simulink model "DataloggerUDP"  (R2015a)
settings: Solver=FixedStepDiscrete  SolverMode=SingleTasking  StartTime=0.0  StopTime=10.0  FixedStep=1e-3  RelTol=1e-3
libraries: mbed_ethernet_udp x3, mbed_lib x2, simulink x1
settings Model: Creator=oh  LastModifiedBy=oh
settings OptimizationCC: OptimizeModelRefInitCode=on  LifeSpan=1
settings HardwareCC: ProdLargestAtomicInteger=Long  ProdLargestAtomicFloat=Double  ProdEndianess=LittleEndian  ProdHWDeviceType=ARM Compatible->ARM Cortex
settings RTWCC: SystemTargetFile=mbed.tlc  TemplateMakefile=mbed.tmf  Description=Mbed Target (Embedded Target)  TargetLang=C++
settings CodeAppCC: IgnoreCustomStorageClasses=off
settings STFCustomTargetCC: CombineOutputUpdateFcns=on  SupportContinuousTime=off  SupportVariableSizeSignals=off  SystemTargetFile=mbed.tlc
settings ERTTargetCC: SupportContinuousTime=off  SupportVariableSizeSignals=off  ERTCustomFileTemplate=mbed_file_process.tlc

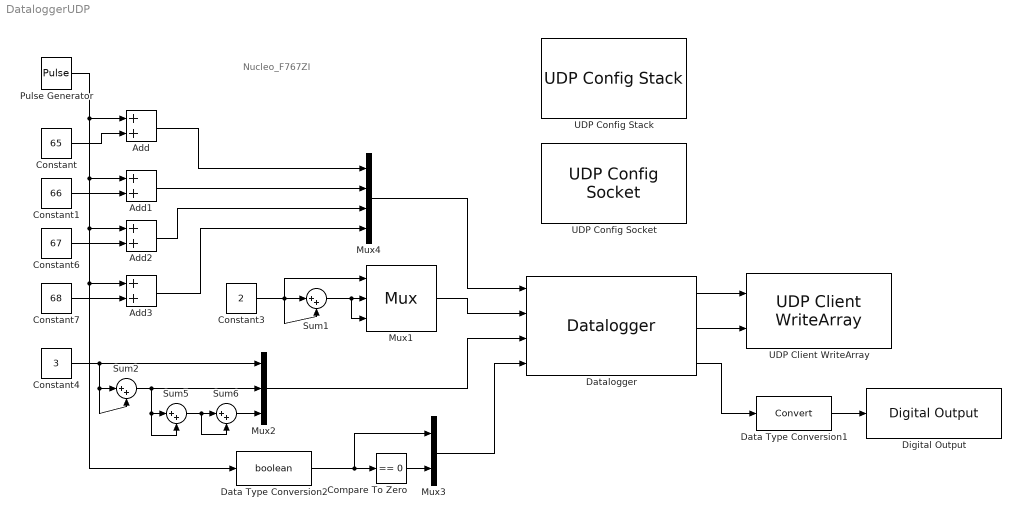
== system DataloggerUDP ==
  note: Nucleo_F767ZI
  Add{,1..3} (4 alike) : Sum  OutDataTypeStr=uint8
  Compare To Zero : simulink/Logic and Bit Operations/Compare To Zero  relop===  OutDataTypeStr=boolean
  Constant : Constant  Value=65
  Constant1 : Constant  Value=66
  Constant3 : Constant  Value=2  OutDataTypeStr=int16
  Constant4 : Constant  Value=3
  Constant6 : Constant  Value=67
  Constant7 : Constant  Value=68
  Data Type Conversion1 : DataTypeConversion
  Data Type Conversion2 : DataTypeConversion  OutDataTypeStr=boolean
  Datalogger : mbed_lib/Utilities/Datalogger  TypeInputPorts={ 'uint8' 4 'int16' 3 'double' 3 'bool' 2 }  TypeOfInputs={'4*uint8' '3*int16' '3*double' '2*bool'}  BufferSize=120  errEn=on  SampleTime=1
  Digital Output : mbed_lib/GPIO/Digital Output  SParameter2=B  SParameter1=0  SParameter3=PullDefault  SampleTime=-1
  Mux1 : Mux  Inputs=3
      settings: DisplayOption=signals
  Mux2 : Mux  Inputs=3
  Mux3 : Mux  Inputs=2
  Mux4 : Mux
  Pulse Generator : DiscretePulseGenerator  PulseType=Time based  Period=5  PulseWidth=50
  Sum{1..2,5..6} (4 alike) : Sum  Inputs=|++
  UDP Client WriteArray : mbed_ethernet_udp/UDP Client WriteArray  sock_ID=1  numData=on  SampleTime=-1
  UDP Config Socket : mbed_ethernet_udp/UDP Config Socket  Priority=1  des_IP='192.168.1.10'  des_port=7195  sock_ID=1
  UDP Config Stack : mbed_ethernet_udp/UDP Config Stack  Priority=0  sDHCP=on  DHCP=1  ip_addr='127.0.0.1'  sub_mask='255.255.255.0'  gateway='0.0.0.0'  DEFAULT_UDP_RECVMBOX_SIZE=8  TCPIP_THREAD_STACKSIZE=1024  TCPIP_THREAD_PRIO=Normal  PBUF_POOL_SIZE=5  TCP_MSS=1460
  wires:
  Sum1/1 -> Mux1/3, Mux1/2
  Sum2/1 -> Mux2/2, Sum5/2, Sum5/1
  Constant3/1 -> Sum1/2, Sum1/1, Mux1/1
  Constant4/1 -> Mux2/1, Sum2/1, Sum2/2
  Sum5/1 -> Sum6/2, Sum6/1
  Data Type Conversion2/1 -> Mux3/1, Compare To Zero/1
  Sum6/1 -> Mux2/3
  Mux2/1 -> Datalogger/3
  Mux1/1 -> Datalogger/2
  Mux3/1 -> Datalogger/4
  Mux4/1 -> Datalogger/1
  Compare To Zero/1 -> Mux3/2
  Datalogger/1 -> UDP Client WriteArray/1
  Datalogger/2 -> UDP Client WriteArray/2
  Datalogger/3 -> Data Type Conversion1/1
  Data Type Conversion1/1 -> Digital Output/1
  Pulse Generator/1 -> Data Type Conversion2/1, Add3/1, Add2/1, Add1/1, Add/1
  Constant/1 -> Add/2
  Constant1/1 -> Add1/2
  Constant6/1 -> Add2/2
  Constant7/1 -> Add3/2
  Add/1 -> Mux4/1
  Add1/1 -> Mux4/2
  Add2/1 -> Mux4/3
  Add3/1 -> Mux4/4
